simulink model "realistic_closed_loop_system"  (R2025b)
settings: Solver=ode5  StartTime=0.0  StopTime=10.0  RelTol=1e-3
values from neighbouring files (symbols this model uses):
  A = [0, 0, 1, 0 ... (first row only)    [inv_pend.m]
  B = [0; 0; (Km*Kg)/(M*Rm*r); (-Km*Kg)/(r*Rm*M*l)]    [inv_pend.m]
  Fa = (pi/2)/6.328    (= 0.248229508027)    [inv_pend.m]
  Fx = 0.456/4.41    (= 0.103401360544)    [inv_pend.m]
  K = lqr(A, B, Q, R)    [inv_pend.m]
  Ts = 0.005    [inv_pend.m]
  Wc = f*2*pi    (= 31.4159265359)    [inv_pend.m]
settings Model: Creator=sm  LastModifiedBy=sm
settings HardwareCC: ProdBitPerLong=64.0  ProdHWDeviceType=Intel->x86-64 (Linux 64)
settings RTWCC: SystemTargetFile=sldrt.tlc  TemplateMakefile=sldrt.tmf  RTWCompilerOptimization=on  Description=Simulink Desktop Real-Time
settings CodeAppCC: MaxIdLength=95.0
settings SimulinkDesktopRealTimeCC: ExtModeTransport=0.0  ExtModeStaticAllocSize=1000000.0  TargetLibSuffix=_sldrt.a  TargetPreCompLibLocation=/usr/local/MATLAB/R2025b/toolbox/sldrt/lib/glnxa64  MultiwordLength=2048.0  DynamicStringBufferSize=256.0  ParMdlRefBuildCompliant=on  PreserveMATLABNamespacesInGeneratedCode=on  SubcomponentCodeInterfacePackaging=Reusable function

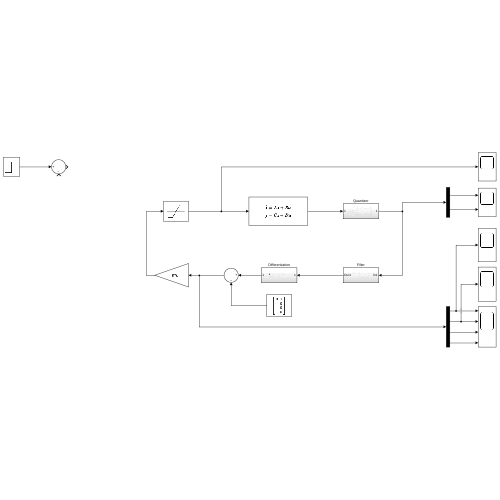
[thumbnail: Simulink's stored preview of the top-level diagram]
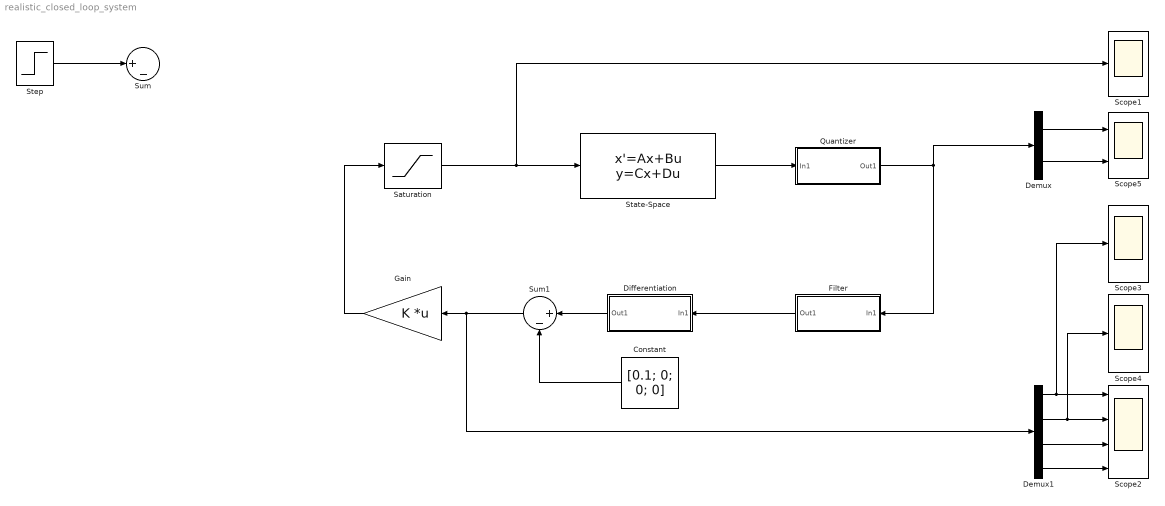
== system realistic_closed_loop_system ==
  Constant : Constant  Value=[0.1; 0; 0; 0]  VectorParams1D=off
  Demux : Demux  Outputs=2
  Demux1 : Demux
  Differentiation : Subsystem
  Filter : Subsystem
  Gain : Gain  Gain=K  Multiplication=Matrix(K*u)
  Quantizer : Subsystem
  Saturation : Saturate  UpperLimit=5  LowerLimit=-5
  Scope1 : Scope
      settings: Title=Voltage [V]  ActiveDisplayYMinimum=-24.163791154276673  ActiveDisplayYMaximum=34.351697914703692  DataLoggingVariableName=step_voltage
  Scope2 : Scope  NumInputPorts=4
      settings: Title=Filtered Anglular Position [rad]  ActiveDisplayYMinimum=-0.64808142081073672  ActiveDisplayYMaximum=0.37740044873205181  DataLoggingVariableName=realistic
  Scope3 : Scope
      settings: Title=Position [m]  ActiveDisplayYMinimum=-1.2457889430215947  ActiveDisplayYMaximum=1.0291530004143326  DataLoggingVariableName=position_sys_cl  DataLoggingSaveFormat=Array
  Scope4 : Scope
      settings: Title=Angular Position [rad]  ActiveDisplayYMinimum=-0.44934447769521407  ActiveDisplayYMaximum=0.27301308046784717  DataLoggingVariableName=angle_step  DataLoggingSaveFormat=Array
  Scope5 : Scope  NumInputPorts=2
      settings: Title=Angular position [rad]  ActiveDisplayYMinimum=-24.163791154276673  ActiveDisplayYMaximum=34.351697914703692  DataLoggingVariableName=step_voltage1
  State-Space : StateSpace  A=A  B=B  C=[1, 0, 0, 0; 0, 1, 0, 0]  D=zeros(2,1)  InitialCondition=[0; 0; 0; 0]
  Step : Step  Time=0  After=3  SampleTime=0
  Sum : Sum  Inputs=|+-
  Sum1 : Sum  Inputs=|+-
  wires:
  Step/1 -> Sum/1
  Demux1/1 -> Scope3/1, Scope2/1
  Demux1/2 -> Scope4/1, Scope2/2
  Demux1/3 -> Scope2/3
  Demux1/4 -> Scope2/4
  Saturation/1 -> Scope1/1, State-Space/1
  Filter/1(Out1) -> Differentiation/1(In1)
  Quantizer/1(Out1) -> Demux/1, Filter/1(In1)
  State-Space/1 -> Quantizer/1(In1)
  Demux/1 -> Scope5/1
  Demux/2 -> Scope5/2
  Gain/1 -> Saturation/1
  Differentiation/1(Out1) -> Sum1/1
  Sum1/1 -> Demux1/1, Gain/1
  Constant/1 -> Sum1/2

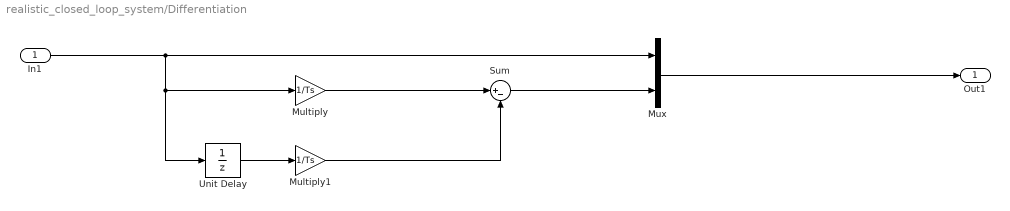
== system realistic_closed_loop_system/Differentiation ==
  In1 : Inport
  Multiply : Gain  Gain=1/Ts
  Multiply1 : Gain  Gain=1/Ts
  Mux : Mux  Inputs=2
  Sum : Sum  Inputs=|+-
  Unit Delay : UnitDelay  InitialCondition=[0; 0]  SampleTime=0.005  HasFrameUpgradeWarning=on
  Out1 : Outport
  wires:
  In1/1 -> Mux/1, Unit Delay/1, Multiply/1
  Unit Delay/1 -> Multiply1/1
  Multiply/1 -> Sum/1
  Multiply1/1 -> Sum/2
  Sum/1 -> Mux/2
  Mux/1 -> Out1/1

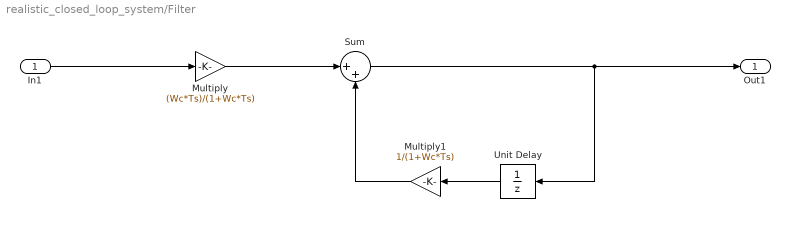
== system realistic_closed_loop_system/Filter ==
  In1 : Inport
  Multiply : Gain  Gain=(Wc*Ts)/(1+Wc*Ts)
  Multiply1 : Gain  Gain=1/(1+Wc*Ts)
  Sum : Sum  Inputs=|++
  Unit Delay : UnitDelay  InitialCondition=[0; 0]  SampleTime=0.005  HasFrameUpgradeWarning=on
  Out1 : Outport
  wires:
  In1/1 -> Multiply/1
  Multiply/1 -> Sum/1
  Sum/1 -> Unit Delay/1, Out1/1
  Multiply1/1 -> Sum/2
  Unit Delay/1 -> Multiply1/1

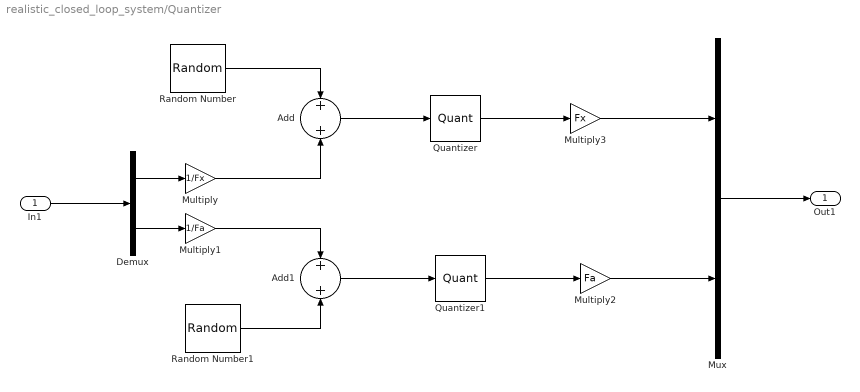
== system realistic_closed_loop_system/Quantizer ==
  In1 : Inport
  Add : Sum
  Add1 : Sum
  Demux : Demux  Outputs=2
  Multiply : Gain  Gain=1/Fx
  Multiply1 : Gain  Gain=1/Fa
  Multiply2 : Gain  Gain=Fa
  Multiply3 : Gain  Gain=Fx
  Mux : Mux  Inputs=2
  Quantizer : Quantizer  QuantizationInterval=20/2^16
  Quantizer1 : Quantizer  QuantizationInterval=20/2^16
  Random Number : RandomNumber  Variance=10^-4  Seed=1  SampleTime=0.005
  Random Number1 : RandomNumber  Variance=10^-4  Seed=2  SampleTime=0.005
  Out1 : Outport
  wires:
  In1/1 -> Demux/1
  Mux/1 -> Out1/1
  Demux/1 -> Multiply/1
  Demux/2 -> Multiply1/1
  Multiply/1 -> Add/2
  Multiply1/1 -> Add1/1
  Add1/1 -> Quantizer1/1
  Multiply2/1 -> Mux/2
  Multiply3/1 -> Mux/1
  Add/1 -> Quantizer/1
  Random Number/1 -> Add/1
  Random Number1/1 -> Add1/2
  Quantizer/1 -> Multiply3/1
  Quantizer1/1 -> Multiply2/1
